simulink model "YawTV_4WD"  (R2025b)
settings: Solver=FixedStepAuto  StartTime=0.0  StopTime=5  FixedStep=1e-3  RelTol=1e-3
settings Model: Creator=nikol  LastModifiedBy=nikol

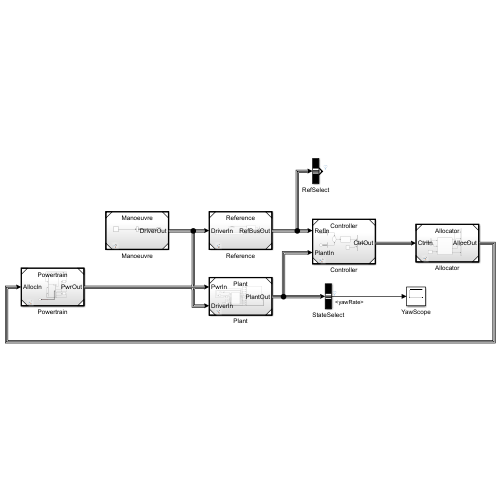
[thumbnail: Simulink's stored preview of the top-level diagram]
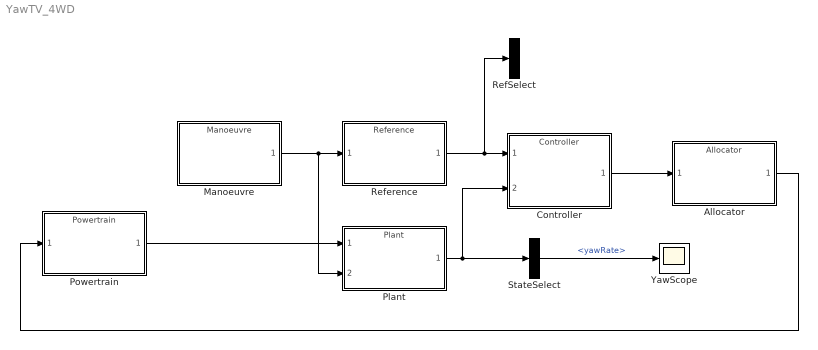
== system YawTV_4WD ==
  Allocator : ModelReference  ModelNameDialog=Allocator  SimulationMode=Normal  ModelReferenceVersion=1.6
  Controller : ModelReference  ModelNameDialog=Controller  SimulationMode=Normal  ModelReferenceVersion=1.6
  Manoeuvre : ModelReference  ModelNameDialog=Manoeuvre  SimulationMode=Normal  ModelReferenceVersion=1.1
  Plant : ModelReference  ModelNameDialog=Plant  SimulationMode=Normal  ModelReferenceVersion=1.18
  Powertrain : ModelReference  ModelNameDialog=Powertrain  SimulationMode=Normal  ModelReferenceVersion=1.6
  RefSelect : BusSelector  OutputSignals=yawRateRef
  Reference : ModelReference  ModelNameDialog=Reference  SimulationMode=Normal  ModelReferenceVersion=1.10
  StateSelect : BusSelector  OutputSignals=yawRate
  YawScope : Scope
      settings: ActiveDisplayYMinimum=-0.039108538353188477  ActiveDisplayYMaximum=0.35197684517869637
  wires:
  Powertrain/1 -> Plant/1
  Reference/1 -> Controller/1, RefSelect/1
  Plant/1 -> Controller/2, StateSelect/1
  Allocator/1 -> Powertrain/1
  Controller/1 -> Allocator/1
  StateSelect/1 -> YawScope/1  "<yawRate>"
  Manoeuvre/1 -> Plant/2, Reference/1
